simulink model "LUT_liver_pancreas_25"  (R2023b)
settings: Solver=FixedStepAuto  StartTime=0  StopTime=10.1  FixedStep=Timegap  RelTol=1e-3
model workspace (MAT data in the model file):
  T1_input = 1.34
(part 1 of 3)
settings Model: Creator=ppxmr2  LastModifiedBy=ppxmr2

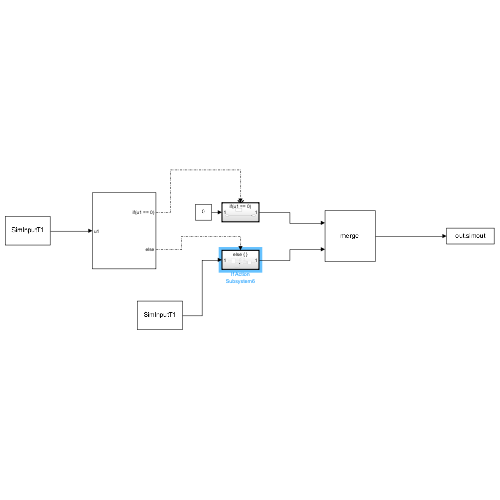
[thumbnail: Simulink's stored preview of the top-level diagram]
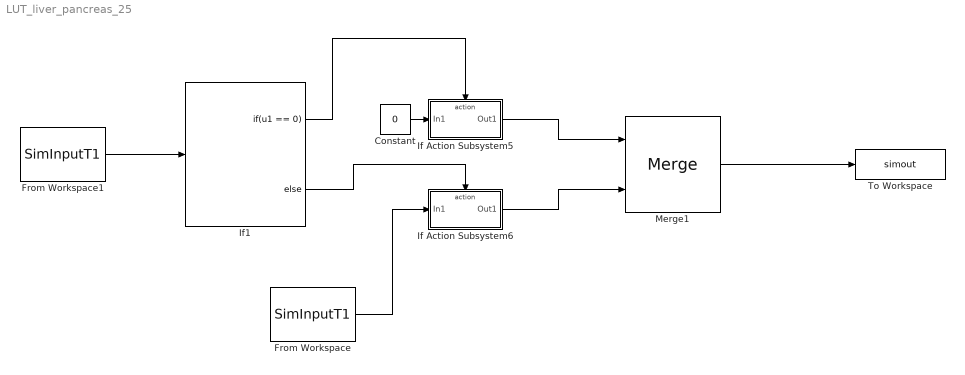
== system LUT_liver_pancreas_25 ==
  Constant : Constant  Value=0
  From Workspace : FromWorkspace  VariableName=SimInputT1  Interpolate=off  OutputAfterFinalValue=Setting to zero
  From Workspace1 : FromWorkspace  VariableName=SimInputT1  Interpolate=off  OutputAfterFinalValue=Setting to zero
  If Action Subsystem5 : Subsystem  TreatAsAtomicUnit=on
  If Action Subsystem6 : Subsystem  TreatAsAtomicUnit=on
  If1 : If  IfExpression=u1 == 0
  Merge1 : Merge
  To Workspace : ToWorkspace  VariableName=simout
  wires:
  From Workspace1/1 -> If1/1
  If1/1 -> If Action Subsystem5/Action
  If1/2 -> If Action Subsystem6/Action
  Constant/1 -> If Action Subsystem5/1(In1)
  If Action Subsystem5/1(Out1) -> Merge1/1
  If Action Subsystem6/1(Out1) -> Merge1/2
  Merge1/1 -> To Workspace/1
  From Workspace/1 -> If Action Subsystem6/1(In1)

== system LUT_liver_pancreas_25/If Action Subsystem5 ==
  In1 : Inport
  Action Port : ActionPort  ActionPortLabel=if(u1 == 0)
  Out1 : Outport
  wires:
  In1/1 -> Out1/1

== system LUT_liver_pancreas_25/If Action Subsystem6 ==
  In1 : Inport
  Action Port : ActionPort  ActionPortLabel=else
  From Workspace1 : FromWorkspace  VariableName=SimInputHR  Interpolate=off  OutputAfterFinalValue=Setting to zero
  If : If  IfExpression=u1 >= 1.495  ElseIfExpressions=u1 >= 0.995
  If Action Subsystem1 : Subsystem  TreatAsAtomicUnit=on
  If Action Subsystem2 : Subsystem  TreatAsAtomicUnit=on
  If Action Subsystem3 : Subsystem  TreatAsAtomicUnit=on
  Merge : Merge  Inputs=3
  Out1 : Outport
  wires:
  Merge/1 -> Out1/1
  From Workspace1/1 -> If/1
  If Action Subsystem1/1(Out1) -> Merge/2
  If Action Subsystem3/1(Out1) -> Merge/3
  In1/1 -> If Action Subsystem2/1(In1), If Action Subsystem1/1(In1), If Action Subsystem3/1(In1)
  If/1 -> If Action Subsystem2/Action
  If/2 -> If Action Subsystem1/Action
  If/3 -> If Action Subsystem3/Action
  If Action Subsystem2/1(Out1) -> Merge/1

== system LUT_liver_pancreas_25/If Action Subsystem6/If Action Subsystem1 ==
  In1 : Inport
  Action Port : ActionPort  ActionPortLabel=elseif(u1 >= 0.995)
  From Workspace2 : FromWorkspace  VariableName=SimInputHR  Interpolate=off  OutputAfterFinalValue=Setting to zero
  If Action Subsystem5 : Subsystem  TreatAsAtomicUnit=on
  If Action Subsystem6 : Subsystem  TreatAsAtomicUnit=on
  If Action Subsystem7 : Subsystem  TreatAsAtomicUnit=on
  If Action Subsystem8 : Subsystem  TreatAsAtomicUnit=on
  If Action Subsystem9 : Subsystem  TreatAsAtomicUnit=on
  If1 : If  IfExpression=u1 >= 1.395  ElseIfExpressions=u1 >= 1.295, u1 >= 1.195, u1 >= 1.095
  Merge1 : Merge  Inputs=5
  Out1 : Outport
  wires:
  In1/1 -> If Action Subsystem7/1(In2), If Action Subsystem8/1(In1), If Action Subsystem9/1(In1), If Action Subsystem5/1(In1), If Action Subsystem6/1(In1)
  From Workspace2/1 -> If1/1
  If Action Subsystem9/1(Out1) -> Merge1/1
  If Action Subsystem6/1(Out1) -> Merge1/5
  If Action Subsystem8/1(Out1) -> Merge1/2
  If Action Subsystem5/1(Out1) -> Merge1/4
  If1/4 -> If Action Subsystem5/Action
  If1/2 -> If Action Subsystem8/Action
  If1/3 -> If Action Subsystem7/Action
  If Action Subsystem7/1(Out2) -> Merge1/3
  If1/5 -> If Action Subsystem6/Action
  If1/1 -> If Action Subsystem9/Action
  Merge1/1 -> Out1/1

== system LUT_liver_pancreas_25/If Action Subsystem6/If Action Subsystem2 ==
  In1 : Inport
  Action Port : ActionPort  ActionPortLabel=if(u1 >= 1.495)
  From Workspace2 : FromWorkspace  VariableName=SimInputHR  Interpolate=off  OutputAfterFinalValue=Setting to zero
  If Action Subsystem5 : Subsystem  TreatAsAtomicUnit=on
  If Action Subsystem6 : Subsystem  TreatAsAtomicUnit=on
  If Action Subsystem7 : Subsystem  TreatAsAtomicUnit=on
  If Action Subsystem8 : Subsystem  TreatAsAtomicUnit=on
  If Action Subsystem9 : Subsystem  TreatAsAtomicUnit=on
  If1 : If  IfExpression=u1 >= 1.895  ElseIfExpressions=u1 >= 1.795, u1 >= 1.695, u1 >= 1.595
  Merge1 : Merge  Inputs=5
  Out1 : Outport
  wires:
  In1/1 -> If Action Subsystem9/1(In1), If Action Subsystem8/1(In1), If Action Subsystem7/1(In1), If Action Subsystem5/1(In1), If Action Subsystem6/1(In1)
  From Workspace2/1 -> If1/1
  If Action Subsystem9/1(Out1) -> Merge1/1
  If1/4 -> If Action Subsystem5/Action
  If1/2 -> If Action Subsystem8/Action
  If1/3 -> If Action Subsystem7/Action
  If1/5 -> If Action Subsystem6/Action
  If1/1 -> If Action Subsystem9/Action
  Merge1/1 -> Out1/1
  If Action Subsystem8/1(Out1) -> Merge1/2
  If Action Subsystem7/1(Out1) -> Merge1/3
  If Action Subsystem6/1(Out1) -> Merge1/5
  If Action Subsystem5/1(Out1) -> Merge1/4

== system LUT_liver_pancreas_25/If Action Subsystem6/If Action Subsystem3 ==
  In1 : Inport
  Action Port : ActionPort  ActionPortLabel=else
  From Workspace2 : FromWorkspace  VariableName=SimInputHR  Interpolate=off  OutputAfterFinalValue=Setting to zero
  If Action Subsystem5 : Subsystem  TreatAsAtomicUnit=on
  If Action Subsystem6 : Subsystem  TreatAsAtomicUnit=on
  If Action Subsystem7 : Subsystem  TreatAsAtomicUnit=on
  If Action Subsystem8 : Subsystem  TreatAsAtomicUnit=on
  If Action Subsystem9 : Subsystem  TreatAsAtomicUnit=on
  If1 : If  IfExpression=u1 >= 0.895  ElseIfExpressions=u1 >= 0.795, u1 >= 0.695, u1 >= 0595
  Merge1 : Merge  Inputs=5
  Out1 : Outport
  wires:
  In1/1 -> If Action Subsystem8/1(In1), If Action Subsystem9/1(In2), If Action Subsystem7/1(In1), If Action Subsystem5/1(In1), If Action Subsystem6/1(In1)
  From Workspace2/1 -> If1/1
  If Action Subsystem9/1(Out2) -> Merge1/1
  If Action Subsystem6/1(Out1) -> Merge1/5
  If Action Subsystem8/1(Out1) -> Merge1/2
  If Action Subsystem5/1(Out1) -> Merge1/4
  If1/4 -> If Action Subsystem5/Action
  If1/2 -> If Action Subsystem8/Action
  If1/3 -> If Action Subsystem7/Action
  If Action Subsystem7/1(Out1) -> Merge1/3
  If1/5 -> If Action Subsystem6/Action
  If1/1 -> If Action Subsystem9/Action
  Merge1/1 -> Out1/1

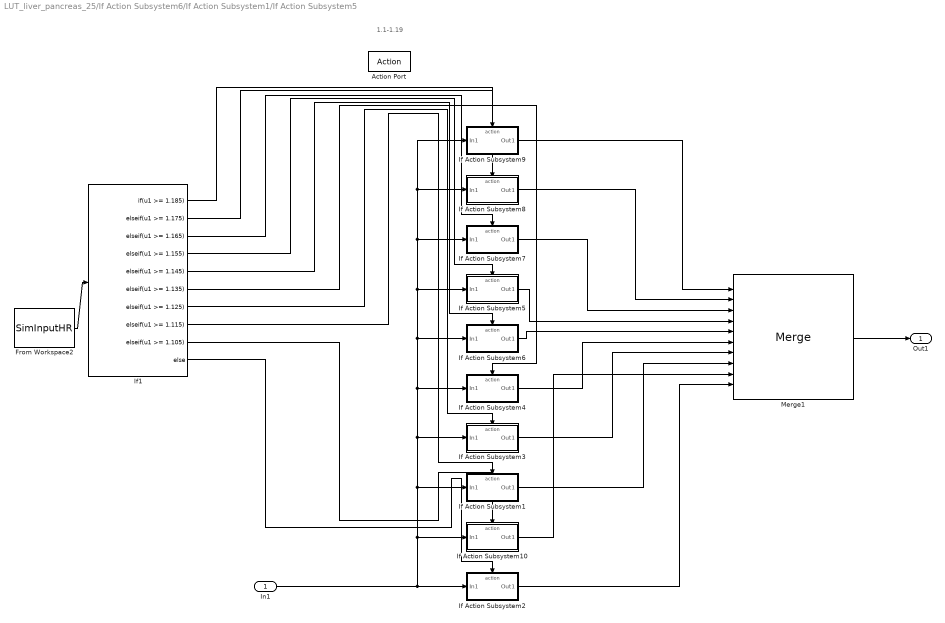
== system LUT_liver_pancreas_25/If Action Subsystem6/If Action Subsystem1/If Action Subsystem5 ==
  note: 1.1-1.19
  In1 : Inport
  Action Port : ActionPort  ActionPortLabel=elseif( u1 >= 1.095)
  From Workspace2 : FromWorkspace  VariableName=SimInputHR  Interpolate=off  OutputAfterFinalValue=Setting to zero
  If Action Subsystem1 : Subsystem  TreatAsAtomicUnit=on
  If Action Subsystem10 : Subsystem  TreatAsAtomicUnit=on
  If Action Subsystem2 : Subsystem  TreatAsAtomicUnit=on
  If Action Subsystem3 : Subsystem  TreatAsAtomicUnit=on
  If Action Subsystem4 : Subsystem  TreatAsAtomicUnit=on
  If Action Subsystem5 : Subsystem  TreatAsAtomicUnit=on
  If Action Subsystem6 : Subsystem  TreatAsAtomicUnit=on
  If Action Subsystem7 : Subsystem  TreatAsAtomicUnit=on
  If Action Subsystem8 : Subsystem  TreatAsAtomicUnit=on
  If Action Subsystem9 : Subsystem  TreatAsAtomicUnit=on
  If1 : If  IfExpression=u1 >= 1.185  ElseIfExpressions=u1 >= 1.175, u1 >= 1.165, u1 >= 1.155, u1 >= 1.145, u1 >= 1.135, u1 >= 1.125, u1 >= 1.115, u1 >= 1.105
  Merge1 : Merge  Inputs=10
  Out1 : Outport
  wires:
  If1/10 -> If Action Subsystem2/Action
  If Action Subsystem4/1(Out1) -> Merge1/6
  From Workspace2/1 -> If1/1
  If Action Subsystem6/1(Out1) -> Merge1/5
  Merge1/1 -> Out1/1
  If1/8 -> If Action Subsystem1/Action
  If Action Subsystem3/1(Out1) -> Merge1/7
  In1/1 -> If Action Subsystem1/1(In1), If Action Subsystem3/1(In1), If Action Subsystem4/1(In1), If Action Subsystem7/1(In1), If Action Subsystem8/1(In1), If Action Subsystem9/1(In1), If Action Subsystem5/1(In1), If Action Subsystem6/1(In1), If Action Subsystem10/1(In1), If Action Subsystem2/1(In1)
  If1/6 -> If Action Subsystem4/Action
  If Action Subsystem1/1(Out1) -> Merge1/8
  If1/4 -> If Action Subsystem5/Action
  If Action Subsystem8/1(Out1) -> Merge1/2
  If1/5 -> If Action Subsystem6/Action
  If Action Subsystem7/1(Out1) -> Merge1/3
  If1/3 -> If Action Subsystem7/Action
  If1/7 -> If Action Subsystem3/Action
  If Action Subsystem5/1(Out1) -> Merge1/4
  If Action Subsystem2/1(Out1) -> Merge1/10
  If1/2 -> If Action Subsystem8/Action
  If1/1 -> If Action Subsystem9/Action
  If Action Subsystem9/1(Out1) -> Merge1/1
  If1/9 -> If Action Subsystem10/Action
  If Action Subsystem10/1(Out1) -> Merge1/9

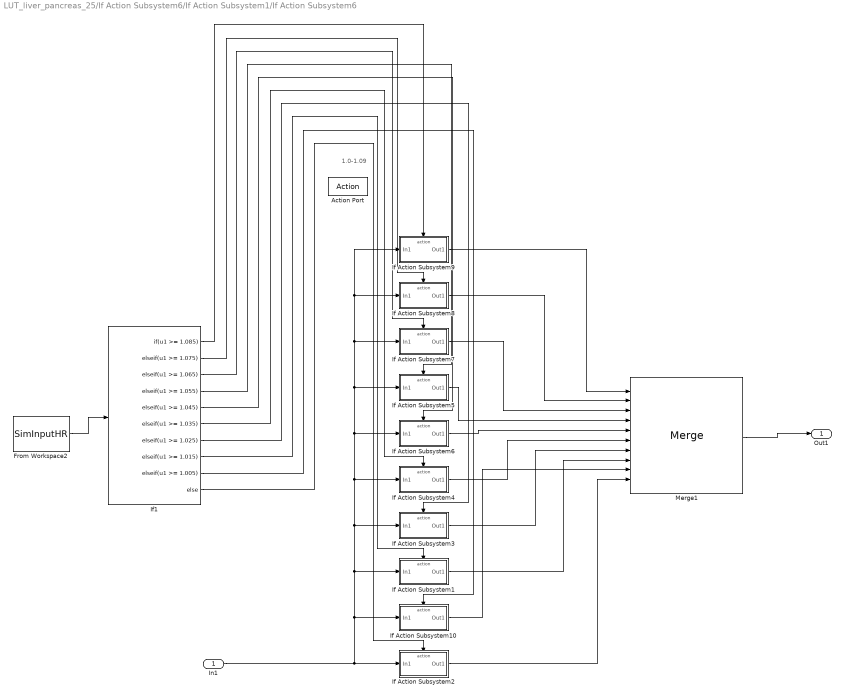
== system LUT_liver_pancreas_25/If Action Subsystem6/If Action Subsystem1/If Action Subsystem6 ==
  note: 1.0-1.09
  In1 : Inport
  Action Port : ActionPort  ActionPortLabel=else
  From Workspace2 : FromWorkspace  VariableName=SimInputHR  Interpolate=off  OutputAfterFinalValue=Setting to zero
  If Action Subsystem1 : Subsystem  TreatAsAtomicUnit=on
  If Action Subsystem10 : Subsystem  TreatAsAtomicUnit=on
  If Action Subsystem2 : Subsystem  TreatAsAtomicUnit=on
  If Action Subsystem3 : Subsystem  TreatAsAtomicUnit=on
  If Action Subsystem4 : Subsystem  TreatAsAtomicUnit=on
  If Action Subsystem5 : Subsystem  TreatAsAtomicUnit=on
  If Action Subsystem6 : Subsystem  TreatAsAtomicUnit=on
  If Action Subsystem7 : Subsystem  TreatAsAtomicUnit=on
  If Action Subsystem8 : Subsystem  TreatAsAtomicUnit=on
  If Action Subsystem9 : Subsystem  TreatAsAtomicUnit=on
  If1 : If  IfExpression=u1 >= 1.085  ElseIfExpressions=u1 >= 1.075, u1 >= 1.065, u1 >= 1.055, u1 >= 1.045, u1 >= 1.035, u1 >= 1.025, u1 >= 1.015, u1 >= 1.005
  Merge1 : Merge  Inputs=10
  Out1 : Outport
  wires:
  If1/10 -> If Action Subsystem2/Action
  If Action Subsystem4/1(Out1) -> Merge1/6
  From Workspace2/1 -> If1/1
  If Action Subsystem6/1(Out1) -> Merge1/5
  Merge1/1 -> Out1/1
  If1/8 -> If Action Subsystem1/Action
  If Action Subsystem3/1(Out1) -> Merge1/7
  In1/1 -> If Action Subsystem1/1(In1), If Action Subsystem3/1(In1), If Action Subsystem4/1(In1), If Action Subsystem7/1(In1), If Action Subsystem8/1(In1), If Action Subsystem9/1(In1), If Action Subsystem5/1(In1), If Action Subsystem6/1(In1), If Action Subsystem10/1(In1), If Action Subsystem2/1(In1)
  If1/6 -> If Action Subsystem4/Action
  If Action Subsystem1/1(Out1) -> Merge1/8
  If1/4 -> If Action Subsystem5/Action
  If Action Subsystem8/1(Out1) -> Merge1/2
  If1/5 -> If Action Subsystem6/Action
  If Action Subsystem7/1(Out1) -> Merge1/3
  If1/3 -> If Action Subsystem7/Action
  If1/7 -> If Action Subsystem3/Action
  If Action Subsystem5/1(Out1) -> Merge1/4
  If Action Subsystem2/1(Out1) -> Merge1/10
  If1/2 -> If Action Subsystem8/Action
  If1/1 -> If Action Subsystem9/Action
  If Action Subsystem9/1(Out1) -> Merge1/1
  If1/9 -> If Action Subsystem10/Action
  If Action Subsystem10/1(Out1) -> Merge1/9

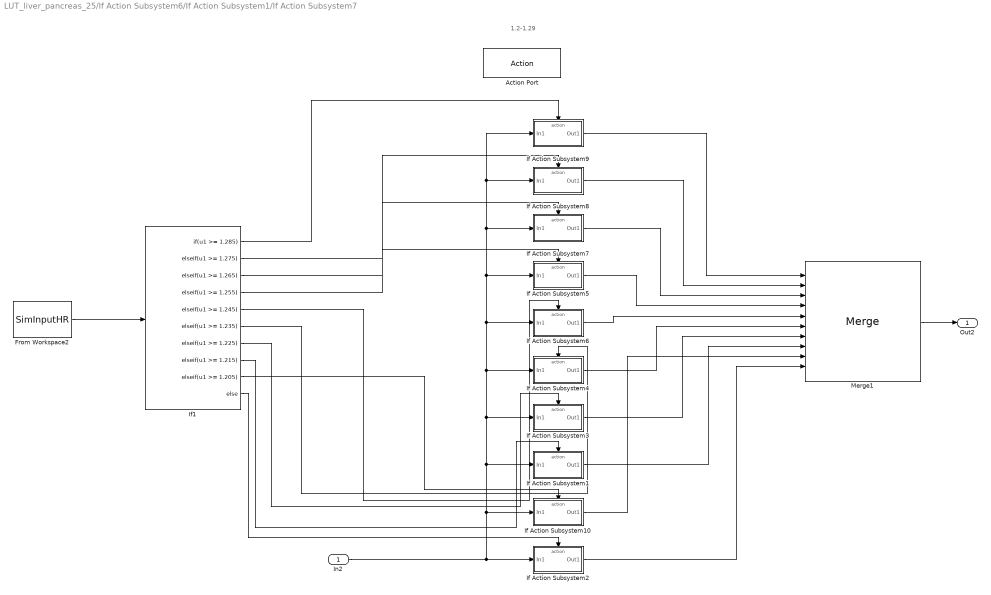
== system LUT_liver_pancreas_25/If Action Subsystem6/If Action Subsystem1/If Action Subsystem7 ==
  note: 1.2-1.29
  In2 : Inport
  Action Port : ActionPort  ActionPortLabel=elseif( u1 >= 1.195)
  From Workspace2 : FromWorkspace  VariableName=SimInputHR  Interpolate=off  OutputAfterFinalValue=Setting to zero
  If Action Subsystem1 : Subsystem  TreatAsAtomicUnit=on
  If Action Subsystem10 : Subsystem  TreatAsAtomicUnit=on
  If Action Subsystem2 : Subsystem  TreatAsAtomicUnit=on
  If Action Subsystem3 : Subsystem  TreatAsAtomicUnit=on
  If Action Subsystem4 : Subsystem  TreatAsAtomicUnit=on
  If Action Subsystem5 : Subsystem  TreatAsAtomicUnit=on
  If Action Subsystem6 : Subsystem  TreatAsAtomicUnit=on
  If Action Subsystem7 : Subsystem  TreatAsAtomicUnit=on
  If Action Subsystem8 : Subsystem  TreatAsAtomicUnit=on
  If Action Subsystem9 : Subsystem  TreatAsAtomicUnit=on
  If1 : If  IfExpression=u1 >= 1.285  ElseIfExpressions=u1 >= 1.275, u1 >= 1.265, u1 >= 1.255, u1 >= 1.245, u1 >= 1.235, u1 >= 1.225, u1 >= 1.215, u1 >= 1.205
  Merge1 : Merge  Inputs=10
  Out2 : Outport
  wires:
  If1/10 -> If Action Subsystem2/Action
  If Action Subsystem4/1(Out1) -> Merge1/6
  From Workspace2/1 -> If1/1
  If Action Subsystem6/1(Out1) -> Merge1/5
  Merge1/1 -> Out2/1
  If1/8 -> If Action Subsystem1/Action
  If Action Subsystem3/1(Out1) -> Merge1/7
  In2/1 -> If Action Subsystem1/1(In1), If Action Subsystem3/1(In1), If Action Subsystem4/1(In1), If Action Subsystem7/1(In1), If Action Subsystem8/1(In1), If Action Subsystem9/1(In1), If Action Subsystem5/1(In1), If Action Subsystem6/1(In1), If Action Subsystem10/1(In1), If Action Subsystem2/1(In1)
  If1/6 -> If Action Subsystem4/Action
  If Action Subsystem1/1(Out1) -> Merge1/8
  If1/4 -> If Action Subsystem5/Action
  If Action Subsystem8/1(Out1) -> Merge1/2
  If1/5 -> If Action Subsystem6/Action
  If Action Subsystem7/1(Out1) -> Merge1/3
  If1/3 -> If Action Subsystem7/Action
  If1/7 -> If Action Subsystem3/Action
  If Action Subsystem5/1(Out1) -> Merge1/4
  If Action Subsystem2/1(Out1) -> Merge1/10
  If1/2 -> If Action Subsystem8/Action
  If1/1 -> If Action Subsystem9/Action
  If Action Subsystem9/1(Out1) -> Merge1/1
  If Action Subsystem10/1(Out1) -> Merge1/9
  If1/9 -> If Action Subsystem10/Action

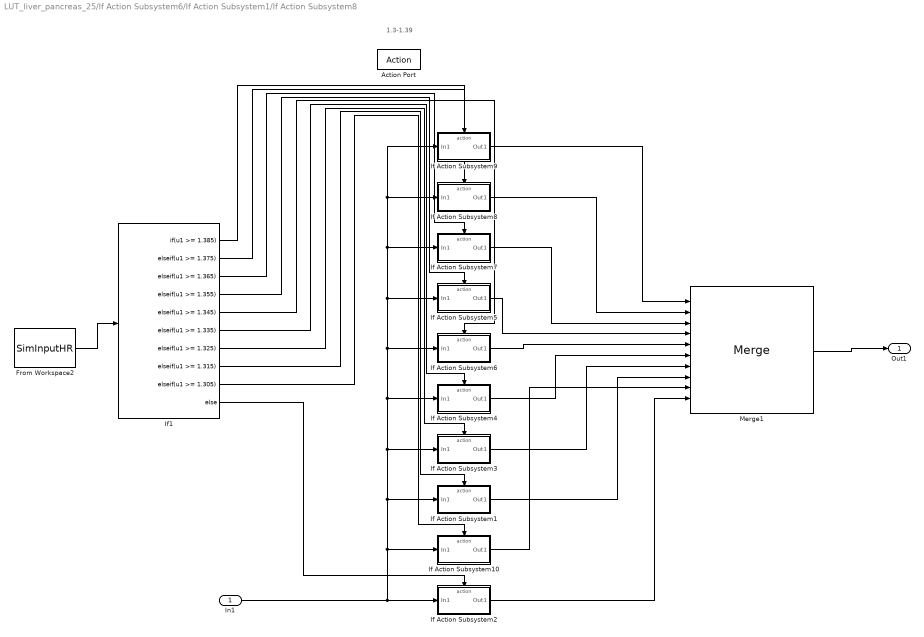
== system LUT_liver_pancreas_25/If Action Subsystem6/If Action Subsystem1/If Action Subsystem8 ==
  note: 1.3-1.39
  In1 : Inport
  Action Port : ActionPort  ActionPortLabel=elseif(u1 >= 1.295)
  From Workspace2 : FromWorkspace  VariableName=SimInputHR  Interpolate=off  OutputAfterFinalValue=Setting to zero
  If Action Subsystem1 : Subsystem  TreatAsAtomicUnit=on
  If Action Subsystem10 : Subsystem  TreatAsAtomicUnit=on
  If Action Subsystem2 : Subsystem  TreatAsAtomicUnit=on
  If Action Subsystem3 : Subsystem  TreatAsAtomicUnit=on
  If Action Subsystem4 : Subsystem  TreatAsAtomicUnit=on
  If Action Subsystem5 : Subsystem  TreatAsAtomicUnit=on
  If Action Subsystem6 : Subsystem  TreatAsAtomicUnit=on
  If Action Subsystem7 : Subsystem  TreatAsAtomicUnit=on
  If Action Subsystem8 : Subsystem  TreatAsAtomicUnit=on
  If Action Subsystem9 : Subsystem  TreatAsAtomicUnit=on
  If1 : If  IfExpression=u1 >= 1.385  ElseIfExpressions=u1 >= 1.375, u1 >= 1.365, u1 >= 1.355, u1 >= 1.345, u1 >= 1.335, u1 >= 1.325, u1 >= 1.315, u1 >= 1.305
  Merge1 : Merge  Inputs=10
  Out1 : Outport
  wires:
  If1/10 -> If Action Subsystem2/Action
  If Action Subsystem4/1(Out1) -> Merge1/6
  From Workspace2/1 -> If1/1
  If Action Subsystem6/1(Out1) -> Merge1/5
  Merge1/1 -> Out1/1
  If1/8 -> If Action Subsystem1/Action
  If Action Subsystem3/1(Out1) -> Merge1/7
  In1/1 -> If Action Subsystem1/1(In1), If Action Subsystem3/1(In1), If Action Subsystem4/1(In1), If Action Subsystem7/1(In1), If Action Subsystem8/1(In1), If Action Subsystem9/1(In1), If Action Subsystem5/1(In1), If Action Subsystem6/1(In1), If Action Subsystem10/1(In1), If Action Subsystem2/1(In1)
  If1/6 -> If Action Subsystem4/Action
  If Action Subsystem1/1(Out1) -> Merge1/8
  If1/4 -> If Action Subsystem5/Action
  If Action Subsystem8/1(Out1) -> Merge1/2
  If1/5 -> If Action Subsystem6/Action
  If Action Subsystem7/1(Out1) -> Merge1/3
  If1/3 -> If Action Subsystem7/Action
  If1/7 -> If Action Subsystem3/Action
  If Action Subsystem5/1(Out1) -> Merge1/4
  If Action Subsystem2/1(Out1) -> Merge1/10
  If1/2 -> If Action Subsystem8/Action
  If1/1 -> If Action Subsystem9/Action
  If Action Subsystem9/1(Out1) -> Merge1/1
  If1/9 -> If Action Subsystem10/Action
  If Action Subsystem10/1(Out1) -> Merge1/9

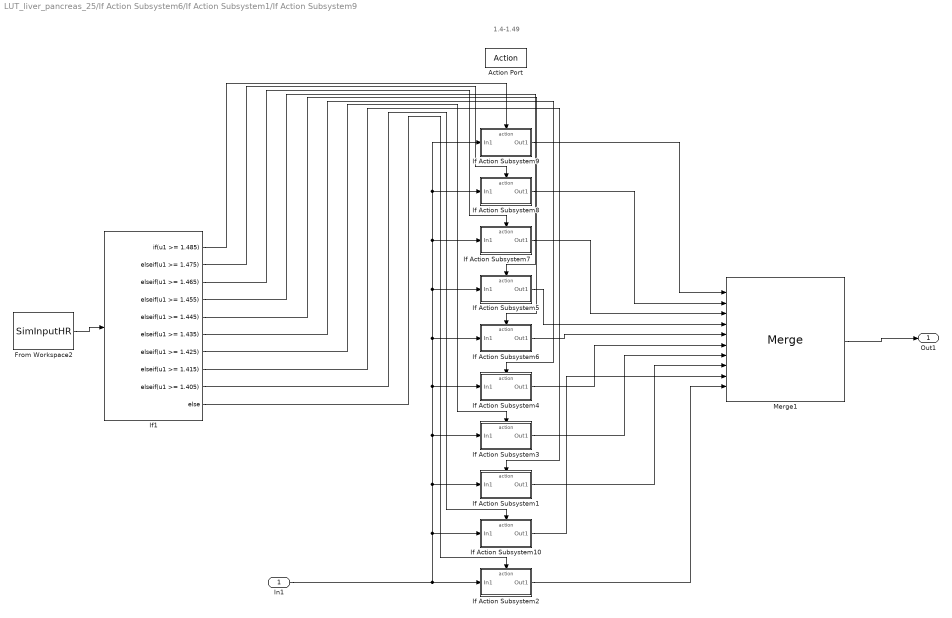
== system LUT_liver_pancreas_25/If Action Subsystem6/If Action Subsystem1/If Action Subsystem9 ==
  note: 1.4-1.49
  In1 : Inport
  Action Port : ActionPort  ActionPortLabel=if(u1 >= 1.395)
  From Workspace2 : FromWorkspace  VariableName=SimInputHR  Interpolate=off  OutputAfterFinalValue=Setting to zero
  If Action Subsystem1 : Subsystem  TreatAsAtomicUnit=on
  If Action Subsystem10 : Subsystem  TreatAsAtomicUnit=on
  If Action Subsystem2 : Subsystem  TreatAsAtomicUnit=on
  If Action Subsystem3 : Subsystem  TreatAsAtomicUnit=on
  If Action Subsystem4 : Subsystem  TreatAsAtomicUnit=on
  If Action Subsystem5 : Subsystem  TreatAsAtomicUnit=on
  If Action Subsystem6 : Subsystem  TreatAsAtomicUnit=on
  If Action Subsystem7 : Subsystem  TreatAsAtomicUnit=on
  If Action Subsystem8 : Subsystem  TreatAsAtomicUnit=on
  If Action Subsystem9 : Subsystem  TreatAsAtomicUnit=on
  If1 : If  IfExpression=u1 >= 1.485  ElseIfExpressions=u1 >= 1.475, u1 >= 1.465, u1 >= 1.455, u1 >= 1.445, u1 >= 1.435, u1 >= 1.425, u1 >= 1.415, u1 >= 1.405
  Merge1 : Merge  Inputs=10
  Out1 : Outport
  wires:
  If1/10 -> If Action Subsystem2/Action
  If Action Subsystem4/1(Out1) -> Merge1/6
  From Workspace2/1 -> If1/1
  If Action Subsystem6/1(Out1) -> Merge1/5
  Merge1/1 -> Out1/1
  If1/8 -> If Action Subsystem1/Action
  If Action Subsystem3/1(Out1) -> Merge1/7
  In1/1 -> If Action Subsystem10/1(In1), If Action Subsystem1/1(In1), If Action Subsystem3/1(In1), If Action Subsystem4/1(In1), If Action Subsystem7/1(In1), If Action Subsystem8/1(In1), If Action Subsystem9/1(In1), If Action Subsystem5/1(In1), If Action Subsystem6/1(In1), If Action Subsystem2/1(In1)
  If1/6 -> If Action Subsystem4/Action
  If Action Subsystem1/1(Out1) -> Merge1/8
  If1/4 -> If Action Subsystem5/Action
  If Action Subsystem8/1(Out1) -> Merge1/2
  If1/5 -> If Action Subsystem6/Action
  If Action Subsystem7/1(Out1) -> Merge1/3
  If1/3 -> If Action Subsystem7/Action
  If1/7 -> If Action Subsystem3/Action
  If Action Subsystem5/1(Out1) -> Merge1/4
  If Action Subsystem2/1(Out1) -> Merge1/10
  If1/2 -> If Action Subsystem8/Action
  If1/1 -> If Action Subsystem9/Action
  If Action Subsystem9/1(Out1) -> Merge1/1
  If1/9 -> If Action Subsystem10/Action
  If Action Subsystem10/1(Out1) -> Merge1/9

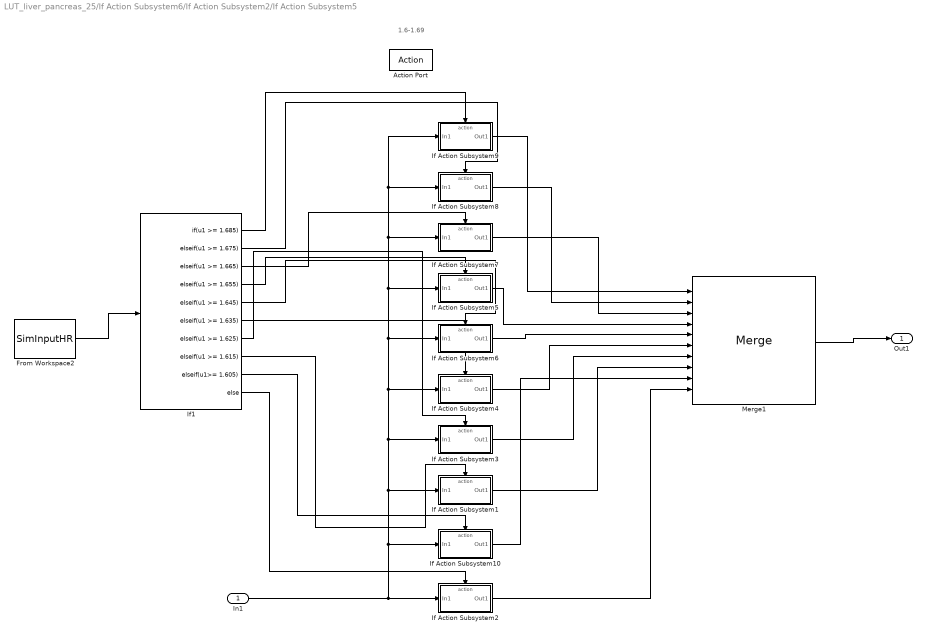
== system LUT_liver_pancreas_25/If Action Subsystem6/If Action Subsystem2/If Action Subsystem5 ==
  note: 1.6-1.69
  In1 : Inport
  Action Port : ActionPort  ActionPortLabel=elseif( u1 >= 1.595)
  From Workspace2 : FromWorkspace  VariableName=SimInputHR  Interpolate=off  OutputAfterFinalValue=Setting to zero
  If Action Subsystem1 : Subsystem  TreatAsAtomicUnit=on
  If Action Subsystem10 : Subsystem  TreatAsAtomicUnit=on
  If Action Subsystem2 : Subsystem  TreatAsAtomicUnit=on
  If Action Subsystem3 : Subsystem  TreatAsAtomicUnit=on
  If Action Subsystem4 : Subsystem  TreatAsAtomicUnit=on
  If Action Subsystem5 : Subsystem  TreatAsAtomicUnit=on
  If Action Subsystem6 : Subsystem  TreatAsAtomicUnit=on
  If Action Subsystem7 : Subsystem  TreatAsAtomicUnit=on
  If Action Subsystem8 : Subsystem  TreatAsAtomicUnit=on
  If Action Subsystem9 : Subsystem  TreatAsAtomicUnit=on
  If1 : If  IfExpression=u1 >= 1.685  ElseIfExpressions=u1 >= 1.675, u1 >= 1.665, u1 >= 1.655, u1 >= 1.645, u1 >= 1.635, u1 >= 1.625, u1 >= 1.615, u1>= 1.605
  Merge1 : Merge  Inputs=10
  Out1 : Outport
  wires:
  If1/2 -> If Action Subsystem8/Action
  If Action Subsystem5/1(Out1) -> Merge1/4
  If1/3 -> If Action Subsystem7/Action
  If Action Subsystem9/1(Out1) -> Merge1/1
  If1/7 -> If Action Subsystem3/Action
  If1/5 -> If Action Subsystem6/Action
  If1/1 -> If Action Subsystem9/Action
  If Action Subsystem4/1(Out1) -> Merge1/6
  If1/10 -> If Action Subsystem2/Action
  If Action Subsystem8/1(Out1) -> Merge1/2
  If1/4 -> If Action Subsystem5/Action
  In1/1 -> If Action Subsystem10/1(In1), If Action Subsystem1/1(In1), If Action Subsystem3/1(In1), If Action Subsystem4/1(In1), If Action Subsystem7/1(In1), If Action Subsystem8/1(In1), If Action Subsystem9/1(In1), If Action Subsystem5/1(In1), If Action Subsystem6/1(In1), If Action Subsystem2/1(In1)
  If Action Subsystem1/1(Out1) -> Merge1/8
  If Action Subsystem2/1(Out1) -> Merge1/10
  If1/8 -> If Action Subsystem1/Action
  If Action Subsystem3/1(Out1) -> Merge1/7
  If1/6 -> If Action Subsystem4/Action
  From Workspace2/1 -> If1/1
  Merge1/1 -> Out1/1
  If Action Subsystem6/1(Out1) -> Merge1/5
  If Action Subsystem7/1(Out1) -> Merge1/3
  If1/9 -> If Action Subsystem10/Action
  If Action Subsystem10/1(Out1) -> Merge1/9

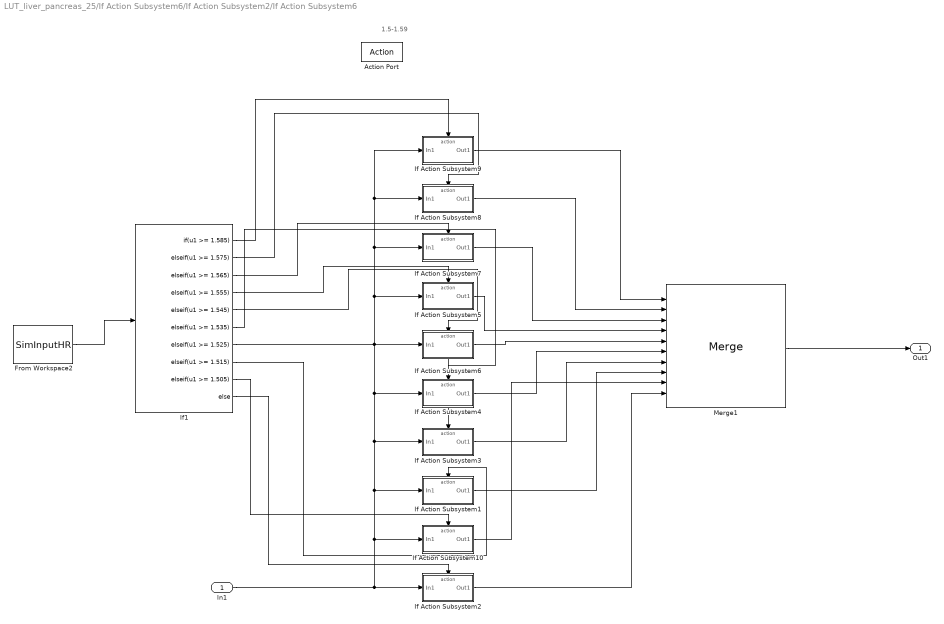
== system LUT_liver_pancreas_25/If Action Subsystem6/If Action Subsystem2/If Action Subsystem6 ==
  note: 1.5-1.59
  In1 : Inport
  Action Port : ActionPort  ActionPortLabel=else
  From Workspace2 : FromWorkspace  VariableName=SimInputHR  Interpolate=off  OutputAfterFinalValue=Setting to zero
  If Action Subsystem1 : Subsystem  TreatAsAtomicUnit=on
  If Action Subsystem10 : Subsystem  TreatAsAtomicUnit=on
  If Action Subsystem2 : Subsystem  TreatAsAtomicUnit=on
  If Action Subsystem3 : Subsystem  TreatAsAtomicUnit=on
  If Action Subsystem4 : Subsystem  TreatAsAtomicUnit=on
  If Action Subsystem5 : Subsystem  TreatAsAtomicUnit=on
  If Action Subsystem6 : Subsystem  TreatAsAtomicUnit=on
  If Action Subsystem7 : Subsystem  TreatAsAtomicUnit=on
  If Action Subsystem8 : Subsystem  TreatAsAtomicUnit=on
  If Action Subsystem9 : Subsystem  TreatAsAtomicUnit=on
  If1 : If  IfExpression=u1 >= 1.585  ElseIfExpressions=u1 >= 1.575, u1 >= 1.565, u1 >= 1.555, u1 >= 1.545, u1 >= 1.535, u1 >= 1.525, u1 >= 1.515, u1 >= 1.505
  Merge1 : Merge  Inputs=10
  Out1 : Outport
  wires:
  If1/2 -> If Action Subsystem8/Action
  If Action Subsystem5/1(Out1) -> Merge1/4
  If1/3 -> If Action Subsystem7/Action
  If Action Subsystem9/1(Out1) -> Merge1/1
  If1/7 -> If Action Subsystem3/Action
  If1/5 -> If Action Subsystem6/Action
  If1/1 -> If Action Subsystem9/Action
  If Action Subsystem4/1(Out1) -> Merge1/6
  If1/10 -> If Action Subsystem2/Action
  If Action Subsystem8/1(Out1) -> Merge1/2
  If1/4 -> If Action Subsystem5/Action
  In1/1 -> If Action Subsystem10/1(In1), If Action Subsystem1/1(In1), If Action Subsystem3/1(In1), If Action Subsystem4/1(In1), If Action Subsystem7/1(In1), If Action Subsystem8/1(In1), If Action Subsystem9/1(In1), If Action Subsystem5/1(In1), If Action Subsystem6/1(In1), If Action Subsystem2/1(In1)
  If Action Subsystem1/1(Out1) -> Merge1/8
  If Action Subsystem2/1(Out1) -> Merge1/10
  If1/8 -> If Action Subsystem1/Action
  If Action Subsystem3/1(Out1) -> Merge1/7
  If1/6 -> If Action Subsystem4/Action
  From Workspace2/1 -> If1/1
  Merge1/1 -> Out1/1
  If Action Subsystem6/1(Out1) -> Merge1/5
  If Action Subsystem7/1(Out1) -> Merge1/3
  If1/9 -> If Action Subsystem10/Action
  If Action Subsystem10/1(Out1) -> Merge1/9

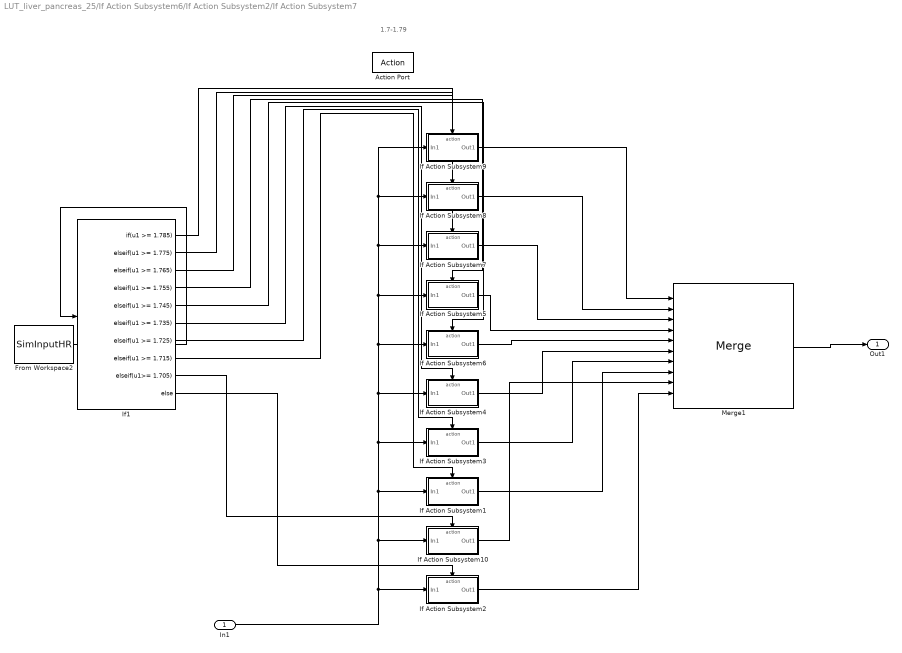
== system LUT_liver_pancreas_25/If Action Subsystem6/If Action Subsystem2/If Action Subsystem7 ==
  note: 1.7-1.79
  In1 : Inport
  Action Port : ActionPort  ActionPortLabel=elseif( u1 >= 1.695)
  From Workspace2 : FromWorkspace  VariableName=SimInputHR  Interpolate=off  OutputAfterFinalValue=Setting to zero
  If Action Subsystem1 : Subsystem  TreatAsAtomicUnit=on
  If Action Subsystem10 : Subsystem  TreatAsAtomicUnit=on
  If Action Subsystem2 : Subsystem  TreatAsAtomicUnit=on
  If Action Subsystem3 : Subsystem  TreatAsAtomicUnit=on
  If Action Subsystem4 : Subsystem  TreatAsAtomicUnit=on
  If Action Subsystem5 : Subsystem  TreatAsAtomicUnit=on
  If Action Subsystem6 : Subsystem  TreatAsAtomicUnit=on
  If Action Subsystem7 : Subsystem  TreatAsAtomicUnit=on
  If Action Subsystem8 : Subsystem  TreatAsAtomicUnit=on
  If Action Subsystem9 : Subsystem  TreatAsAtomicUnit=on
  If1 : If  IfExpression=u1 >= 1.785  ElseIfExpressions=u1 >= 1.775, u1 >= 1.765, u1 >= 1.755, u1 >= 1.745, u1 >= 1.735, u1 >= 1.725, u1 >= 1.715, u1>= 1.705
  Merge1 : Merge  Inputs=10
  Out1 : Outport
  wires:
  If1/2 -> If Action Subsystem8/Action
  If Action Subsystem5/1(Out1) -> Merge1/4
  If1/3 -> If Action Subsystem7/Action
  If Action Subsystem9/1(Out1) -> Merge1/1
  If1/7 -> If Action Subsystem3/Action
  If1/5 -> If Action Subsystem6/Action
  If1/1 -> If Action Subsystem9/Action
  If Action Subsystem4/1(Out1) -> Merge1/6
  If1/10 -> If Action Subsystem2/Action
  If Action Subsystem8/1(Out1) -> Merge1/2
  If1/4 -> If Action Subsystem5/Action
  In1/1 -> If Action Subsystem10/1(In1), If Action Subsystem1/1(In1), If Action Subsystem3/1(In1), If Action Subsystem4/1(In1), If Action Subsystem7/1(In1), If Action Subsystem8/1(In1), If Action Subsystem9/1(In1), If Action Subsystem5/1(In1), If Action Subsystem6/1(In1), If Action Subsystem2/1(In1)
  If Action Subsystem1/1(Out1) -> Merge1/8
  If Action Subsystem2/1(Out1) -> Merge1/10
  If1/8 -> If Action Subsystem1/Action
  If Action Subsystem3/1(Out1) -> Merge1/7
  If1/6 -> If Action Subsystem4/Action
  From Workspace2/1 -> If1/1
  Merge1/1 -> Out1/1
  If Action Subsystem6/1(Out1) -> Merge1/5
  If Action Subsystem7/1(Out1) -> Merge1/3
  If Action Subsystem10/1(Out1) -> Merge1/9
  If1/9 -> If Action Subsystem10/Action

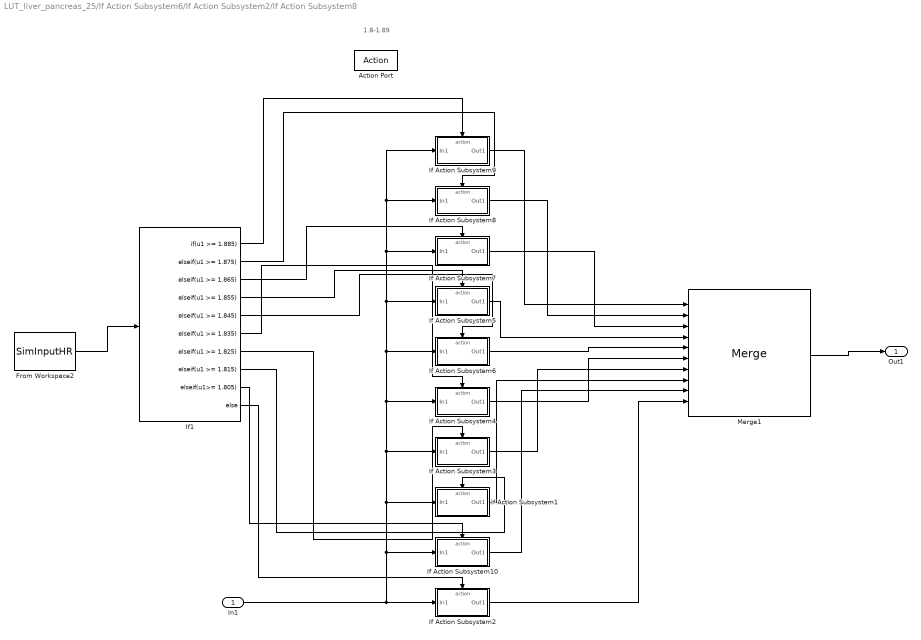
== system LUT_liver_pancreas_25/If Action Subsystem6/If Action Subsystem2/If Action Subsystem8 ==
  note: 1.8-1.89
  In1 : Inport
  Action Port : ActionPort  ActionPortLabel=elseif(u1 >= 1.795)
  From Workspace2 : FromWorkspace  VariableName=SimInputHR  Interpolate=off  OutputAfterFinalValue=Setting to zero
  If Action Subsystem1 : Subsystem  TreatAsAtomicUnit=on
  If Action Subsystem10 : Subsystem  TreatAsAtomicUnit=on
  If Action Subsystem2 : Subsystem  TreatAsAtomicUnit=on
  If Action Subsystem3 : Subsystem  TreatAsAtomicUnit=on
  If Action Subsystem4 : Subsystem  TreatAsAtomicUnit=on
  If Action Subsystem5 : Subsystem  TreatAsAtomicUnit=on
  If Action Subsystem6 : Subsystem  TreatAsAtomicUnit=on
  If Action Subsystem7 : Subsystem  TreatAsAtomicUnit=on
  If Action Subsystem8 : Subsystem  TreatAsAtomicUnit=on
  If Action Subsystem9 : Subsystem  TreatAsAtomicUnit=on
  If1 : If  IfExpression=u1 >= 1.885  ElseIfExpressions=u1 >= 1.875, u1 >= 1.865, u1 >= 1.855, u1 >= 1.845, u1 >= 1.835, u1 >= 1.825, u1 >= 1.815, u1>= 1.805
  Merge1 : Merge  Inputs=10
  Out1 : Outport
  wires:
  If1/2 -> If Action Subsystem8/Action
  If Action Subsystem5/1(Out1) -> Merge1/4
  If1/3 -> If Action Subsystem7/Action
  If Action Subsystem9/1(Out1) -> Merge1/1
  If1/7 -> If Action Subsystem3/Action
  If1/5 -> If Action Subsystem6/Action
  If1/1 -> If Action Subsystem9/Action
  If Action Subsystem4/1(Out1) -> Merge1/6
  If1/10 -> If Action Subsystem2/Action
  If Action Subsystem8/1(Out1) -> Merge1/2
  If1/4 -> If Action Subsystem5/Action
  In1/1 -> If Action Subsystem10/1(In1), If Action Subsystem1/1(In1), If Action Subsystem3/1(In1), If Action Subsystem4/1(In1), If Action Subsystem7/1(In1), If Action Subsystem8/1(In1), If Action Subsystem9/1(In1), If Action Subsystem5/1(In1), If Action Subsystem6/1(In1), If Action Subsystem2/1(In1)
  If Action Subsystem1/1(Out1) -> Merge1/8
  If Action Subsystem2/1(Out1) -> Merge1/10
  If1/8 -> If Action Subsystem1/Action
  If Action Subsystem3/1(Out1) -> Merge1/7
  If1/6 -> If Action Subsystem4/Action
  From Workspace2/1 -> If1/1
  Merge1/1 -> Out1/1
  If Action Subsystem6/1(Out1) -> Merge1/5
  If Action Subsystem7/1(Out1) -> Merge1/3
  If1/9 -> If Action Subsystem10/Action
  If Action Subsystem10/1(Out1) -> Merge1/9

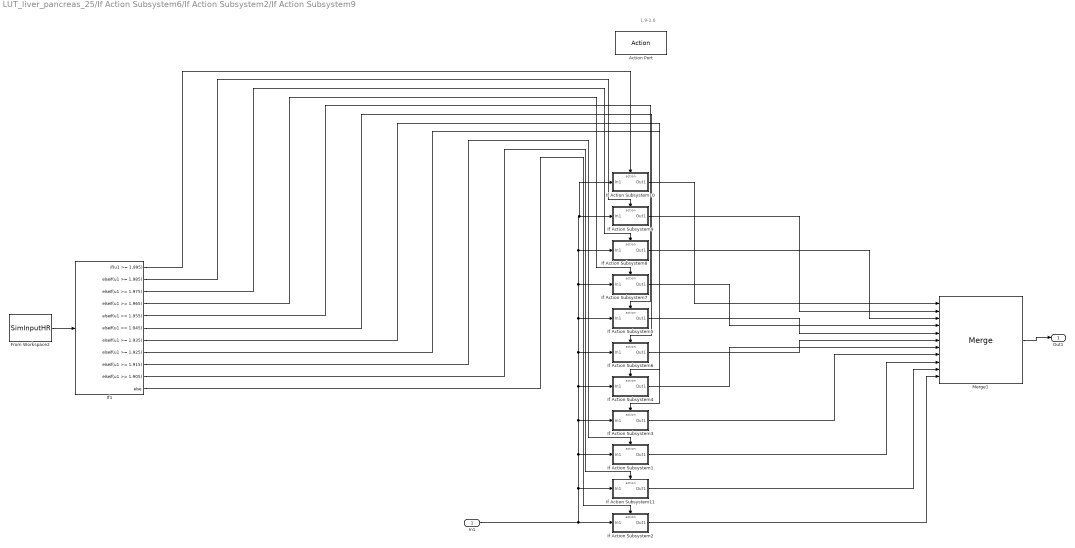
== system LUT_liver_pancreas_25/If Action Subsystem6/If Action Subsystem2/If Action Subsystem9 ==
  note: 1.9-2.0
  In1 : Inport
  Action Port : ActionPort  ActionPortLabel=if(u1 >= 1.895)
  From Workspace2 : FromWorkspace  VariableName=SimInputHR  Interpolate=off  OutputAfterFinalValue=Setting to zero
  If Action Subsystem1 : Subsystem  TreatAsAtomicUnit=on
  If Action Subsystem10 : Subsystem  TreatAsAtomicUnit=on
  If Action Subsystem11 : Subsystem  TreatAsAtomicUnit=on
  If Action Subsystem2 : Subsystem  TreatAsAtomicUnit=on
  If Action Subsystem3 : Subsystem  TreatAsAtomicUnit=on
  If Action Subsystem4 : Subsystem  TreatAsAtomicUnit=on
  If Action Subsystem5 : Subsystem  TreatAsAtomicUnit=on
  If Action Subsystem6 : Subsystem  TreatAsAtomicUnit=on
  If Action Subsystem7 : Subsystem  TreatAsAtomicUnit=on
  If Action Subsystem8 : Subsystem  TreatAsAtomicUnit=on
  If Action Subsystem9 : Subsystem  TreatAsAtomicUnit=on
  If1 : If  IfExpression=u1 >= 1.995  ElseIfExpressions=u1 >= 1.985, u1 >= 1.975, u1 >= 1.965, u1 >= 1.955, u1 >= 1.945, u1 >= 1.935, u1 >= 1.925, u1 >= 1.915, u1 >= 1.905
  Merge1 : Merge  Inputs=11
  Out1 : Outport
  wires:
  Merge1/1 -> Out1/1
  From Workspace2/1 -> If1/1
  If1/2 -> If Action Subsystem9/Action
  If1/3 -> If Action Subsystem8/Action
  If1/4 -> If Action Subsystem7/Action
  If1/5 -> If Action Subsystem5/Action
  If1/6 -> If Action Subsystem6/Action
  If1/7 -> If Action Subsystem4/Action
  If1/8 -> If Action Subsystem3/Action
  If1/9 -> If Action Subsystem1/Action
  If1/11 -> If Action Subsystem2/Action
  If Action Subsystem9/1(Out1) -> Merge1/2
  If Action Subsystem8/1(Out1) -> Merge1/3
  If Action Subsystem7/1(Out1) -> Merge1/4
  If Action Subsystem5/1(Out1) -> Merge1/5
  If Action Subsystem6/1(Out1) -> Merge1/6
  If Action Subsystem4/1(Out1) -> Merge1/7
  If Action Subsystem3/1(Out1) -> Merge1/8
  If Action Subsystem2/1(Out1) -> Merge1/11
  If Action Subsystem1/1(Out1) -> Merge1/9
  In1/1 -> If Action Subsystem1/1(In1), If Action Subsystem3/1(In1), If Action Subsystem4/1(In1), If Action Subsystem7/1(In1), If Action Subsystem8/1(In1), If Action Subsystem10/1(In1), If Action Subsystem9/1(In1), If Action Subsystem5/1(In1), If Action Subsystem6/1(In1), If Action Subsystem11/1(In1), If Action Subsystem2/1(In1)
  If1/1 -> If Action Subsystem10/Action
  If Action Subsystem10/1(Out1) -> Merge1/1
  If1/10 -> If Action Subsystem11/Action
  If Action Subsystem11/1(Out1) -> Merge1/10

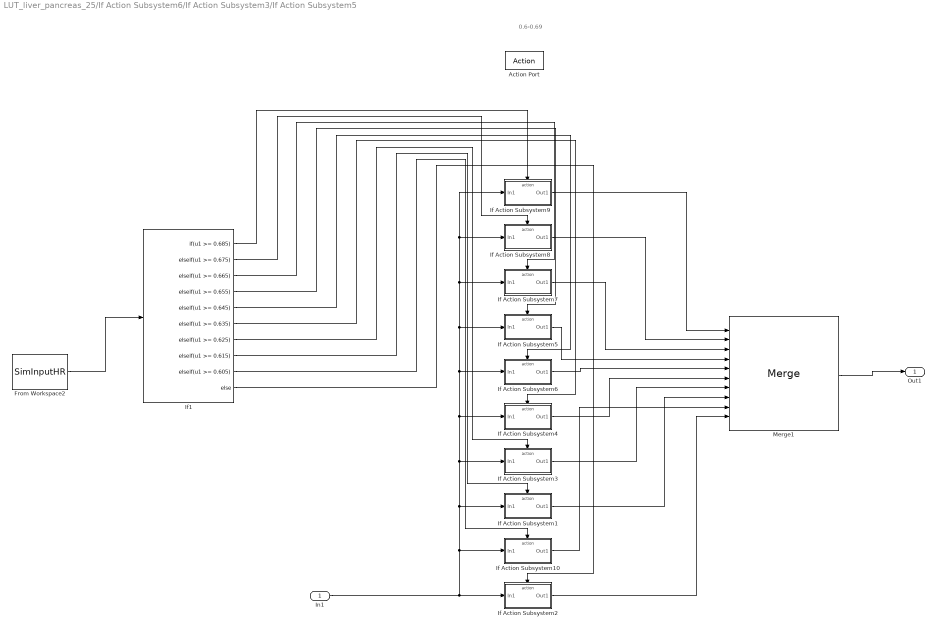
== system LUT_liver_pancreas_25/If Action Subsystem6/If Action Subsystem3/If Action Subsystem5 ==
  note: 0.6-0.69
  In1 : Inport
  Action Port : ActionPort  ActionPortLabel=elseif( u1 >= 0595)
  From Workspace2 : FromWorkspace  VariableName=SimInputHR  Interpolate=off  OutputAfterFinalValue=Setting to zero
  If Action Subsystem1 : Subsystem  TreatAsAtomicUnit=on
  If Action Subsystem10 : Subsystem  TreatAsAtomicUnit=on
  If Action Subsystem2 : Subsystem  TreatAsAtomicUnit=on
  If Action Subsystem3 : Subsystem  TreatAsAtomicUnit=on
  If Action Subsystem4 : Subsystem  TreatAsAtomicUnit=on
  If Action Subsystem5 : Subsystem  TreatAsAtomicUnit=on
  If Action Subsystem6 : Subsystem  TreatAsAtomicUnit=on
  If Action Subsystem7 : Subsystem  TreatAsAtomicUnit=on
  If Action Subsystem8 : Subsystem  TreatAsAtomicUnit=on
  If Action Subsystem9 : Subsystem  TreatAsAtomicUnit=on
  If1 : If  IfExpression=u1 >= 0.685  ElseIfExpressions=u1 >= 0.675, u1 >= 0.665, u1 >= 0.655, u1 >= 0.645, u1 >= 0.635, u1 >= 0.625, u1 >= 0.615, u1 >= 0.605
  Merge1 : Merge  Inputs=10
  Out1 : Outport
  wires:
  If1/10 -> If Action Subsystem2/Action
  If Action Subsystem4/1(Out1) -> Merge1/6
  From Workspace2/1 -> If1/1
  If Action Subsystem6/1(Out1) -> Merge1/5
  Merge1/1 -> Out1/1
  If1/8 -> If Action Subsystem1/Action
  If Action Subsystem3/1(Out1) -> Merge1/7
  In1/1 -> If Action Subsystem1/1(In1), If Action Subsystem3/1(In1), If Action Subsystem4/1(In1), If Action Subsystem7/1(In1), If Action Subsystem8/1(In1), If Action Subsystem9/1(In1), If Action Subsystem5/1(In1), If Action Subsystem6/1(In1), If Action Subsystem10/1(In1), If Action Subsystem2/1(In1)
  If1/6 -> If Action Subsystem4/Action
  If Action Subsystem1/1(Out1) -> Merge1/8
  If1/4 -> If Action Subsystem5/Action
  If Action Subsystem8/1(Out1) -> Merge1/2
  If1/5 -> If Action Subsystem6/Action
  If Action Subsystem7/1(Out1) -> Merge1/3
  If1/3 -> If Action Subsystem7/Action
  If1/7 -> If Action Subsystem3/Action
  If Action Subsystem5/1(Out1) -> Merge1/4
  If Action Subsystem2/1(Out1) -> Merge1/10
  If1/2 -> If Action Subsystem8/Action
  If1/1 -> If Action Subsystem9/Action
  If Action Subsystem9/1(Out1) -> Merge1/1
  If Action Subsystem10/1(Out1) -> Merge1/9
  If1/9 -> If Action Subsystem10/Action

== system LUT_liver_pancreas_25/If Action Subsystem6/If Action Subsystem3/If Action Subsystem6 ==
  note: 0.5-0.59
  In1 : Inport
  Action Port : ActionPort  ActionPortLabel=else
  From Workspace2 : FromWorkspace  VariableName=SimInputHR  Interpolate=off  OutputAfterFinalValue=Setting to zero
  If Action Subsystem1 : Subsystem  TreatAsAtomicUnit=on
  If Action Subsystem10 : Subsystem  TreatAsAtomicUnit=on
  If Action Subsystem2 : Subsystem  TreatAsAtomicUnit=on
  If Action Subsystem3 : Subsystem  TreatAsAtomicUnit=on
  If Action Subsystem4 : Subsystem  TreatAsAtomicUnit=on
  If Action Subsystem5 : Subsystem  TreatAsAtomicUnit=on
  If Action Subsystem6 : Subsystem  TreatAsAtomicUnit=on
  If Action Subsystem7 : Subsystem  TreatAsAtomicUnit=on
  If Action Subsystem8 : Subsystem  TreatAsAtomicUnit=on
  If Action Subsystem9 : Subsystem  TreatAsAtomicUnit=on
  If1 : If  IfExpression=u1 >= 0.585  ElseIfExpressions=u1 >= 0.575, u1 >= 0.565, u1 >= 0.555, u1 >= 0.545, u1 >= 0.535, u1 >= 0.525, u1 >= 0.515, u1 >= 0.505
  Merge1 : Merge  Inputs=10
  Out1 : Outport
  wires:
  If1/10 -> If Action Subsystem2/Action
  If Action Subsystem4/1(Out1) -> Merge1/6
  From Workspace2/1 -> If1/1
  If Action Subsystem6/1(Out1) -> Merge1/5
  Merge1/1 -> Out1/1
  If1/8 -> If Action Subsystem1/Action
  If Action Subsystem3/1(Out1) -> Merge1/7
  In1/1 -> If Action Subsystem1/1(In1), If Action Subsystem3/1(In1), If Action Subsystem4/1(In1), If Action Subsystem7/1(In1), If Action Subsystem8/1(In1), If Action Subsystem9/1(In1), If Action Subsystem5/1(In1), If Action Subsystem6/1(In1), If Action Subsystem10/1(In1), If Action Subsystem2/1(In1)
  If1/6 -> If Action Subsystem4/Action
  If Action Subsystem1/1(Out1) -> Merge1/8
  If1/4 -> If Action Subsystem5/Action
  If Action Subsystem8/1(Out1) -> Merge1/2
  If1/5 -> If Action Subsystem6/Action
  If Action Subsystem7/1(Out1) -> Merge1/3
  If1/3 -> If Action Subsystem7/Action
  If1/7 -> If Action Subsystem3/Action
  If Action Subsystem5/1(Out1) -> Merge1/4
  If Action Subsystem2/1(Out1) -> Merge1/10
  If1/2 -> If Action Subsystem8/Action
  If1/1 -> If Action Subsystem9/Action
  If Action Subsystem9/1(Out1) -> Merge1/1
  If Action Subsystem10/1(Out1) -> Merge1/9
  If1/9 -> If Action Subsystem10/Action

== system LUT_liver_pancreas_25/If Action Subsystem6/If Action Subsystem3/If Action Subsystem7 ==
  note: 0.7-0.79
  In1 : Inport
  Action Port : ActionPort  ActionPortLabel=elseif( u1 >= 0.695)
  From Workspace2 : FromWorkspace  VariableName=SimInputHR  Interpolate=off  OutputAfterFinalValue=Setting to zero
  If Action Subsystem1 : Subsystem  TreatAsAtomicUnit=on
  If Action Subsystem10 : Subsystem  TreatAsAtomicUnit=on
  If Action Subsystem2 : Subsystem  TreatAsAtomicUnit=on
  If Action Subsystem3 : Subsystem  TreatAsAtomicUnit=on
  If Action Subsystem4 : Subsystem  TreatAsAtomicUnit=on
  If Action Subsystem5 : Subsystem  TreatAsAtomicUnit=on
  If Action Subsystem6 : Subsystem  TreatAsAtomicUnit=on
  If Action Subsystem7 : Subsystem  TreatAsAtomicUnit=on
  If Action Subsystem8 : Subsystem  TreatAsAtomicUnit=on
  If Action Subsystem9 : Subsystem  TreatAsAtomicUnit=on
  If1 : If  IfExpression=u1 >= 0.785  ElseIfExpressions=u1 >= 0.775, u1 >= 0.765, u1 >= 0.755, u1 >= 0.745, u1 >= 0.735, u1 >= 0.725, u1 >= 0.715, u1 >= 0.705
  Merge1 : Merge  Inputs=10
  Out1 : Outport
  wires:
  If1/10 -> If Action Subsystem2/Action
  If Action Subsystem4/1(Out1) -> Merge1/6
  From Workspace2/1 -> If1/1
  If Action Subsystem6/1(Out1) -> Merge1/5
  Merge1/1 -> Out1/1
  If1/8 -> If Action Subsystem1/Action
  If Action Subsystem3/1(Out1) -> Merge1/7
  In1/1 -> If Action Subsystem1/1(In1), If Action Subsystem3/1(In1), If Action Subsystem4/1(In1), If Action Subsystem7/1(In1), If Action Subsystem8/1(In1), If Action Subsystem9/1(In1), If Action Subsystem5/1(In1), If Action Subsystem6/1(In1), If Action Subsystem10/1(In1), If Action Subsystem2/1(In1)
  If1/6 -> If Action Subsystem4/Action
  If Action Subsystem1/1(Out1) -> Merge1/8
  If1/4 -> If Action Subsystem5/Action
  If Action Subsystem8/1(Out1) -> Merge1/2
  If1/5 -> If Action Subsystem6/Action
  If Action Subsystem7/1(Out1) -> Merge1/3
  If1/3 -> If Action Subsystem7/Action
  If1/7 -> If Action Subsystem3/Action
  If Action Subsystem5/1(Out1) -> Merge1/4
  If Action Subsystem2/1(Out1) -> Merge1/10
  If1/2 -> If Action Subsystem8/Action
  If1/1 -> If Action Subsystem9/Action
  If Action Subsystem9/1(Out1) -> Merge1/1
  If1/9 -> If Action Subsystem10/Action
  If Action Subsystem10/1(Out1) -> Merge1/9

== system LUT_liver_pancreas_25/If Action Subsystem6/If Action Subsystem3/If Action Subsystem8 ==
  note: 0.8-0.89
  In1 : Inport
  Action Port : ActionPort  ActionPortLabel=elseif(u1 >= 0.795)
  From Workspace2 : FromWorkspace  VariableName=SimInputHR  Interpolate=off  OutputAfterFinalValue=Setting to zero
  If Action Subsystem1 : Subsystem  TreatAsAtomicUnit=on
  If Action Subsystem10 : Subsystem  TreatAsAtomicUnit=on
  If Action Subsystem2 : Subsystem  TreatAsAtomicUnit=on
  If Action Subsystem3 : Subsystem  TreatAsAtomicUnit=on
  If Action Subsystem4 : Subsystem  TreatAsAtomicUnit=on
  If Action Subsystem5 : Subsystem  TreatAsAtomicUnit=on
  If Action Subsystem6 : Subsystem  TreatAsAtomicUnit=on
  If Action Subsystem7 : Subsystem  TreatAsAtomicUnit=on
  If Action Subsystem8 : Subsystem  TreatAsAtomicUnit=on
  If Action Subsystem9 : Subsystem  TreatAsAtomicUnit=on
  If1 : If  IfExpression=u1 >= 0.885  ElseIfExpressions=u1 >= 0.875, u1 >= 0.865, u1 >= 0.855, u1 >= 0.845, u1 >= 0.835, u1 >= 0.825, u1 >= 0.815, u1 >= 0.805
  Merge1 : Merge  Inputs=10
  Out1 : Outport
  wires:
  If1/10 -> If Action Subsystem2/Action
  If Action Subsystem4/1(Out1) -> Merge1/6
  From Workspace2/1 -> If1/1
  If Action Subsystem6/1(Out1) -> Merge1/5
  Merge1/1 -> Out1/1
  If1/8 -> If Action Subsystem1/Action
  If Action Subsystem3/1(Out1) -> Merge1/7
  In1/1 -> If Action Subsystem1/1(In1), If Action Subsystem3/1(In1), If Action Subsystem4/1(In1), If Action Subsystem7/1(In1), If Action Subsystem8/1(In1), If Action Subsystem9/1(In1), If Action Subsystem5/1(In1), If Action Subsystem6/1(In1), If Action Subsystem10/1(In1), If Action Subsystem2/1(In1)
  If1/6 -> If Action Subsystem4/Action
  If Action Subsystem1/1(Out1) -> Merge1/8
  If1/4 -> If Action Subsystem5/Action
  If Action Subsystem8/1(Out1) -> Merge1/2
  If1/5 -> If Action Subsystem6/Action
  If Action Subsystem7/1(Out1) -> Merge1/3
  If1/3 -> If Action Subsystem7/Action
  If1/7 -> If Action Subsystem3/Action
  If Action Subsystem5/1(Out1) -> Merge1/4
  If Action Subsystem2/1(Out1) -> Merge1/10
  If1/2 -> If Action Subsystem8/Action
  If1/1 -> If Action Subsystem9/Action
  If Action Subsystem9/1(Out1) -> Merge1/1
  If1/9 -> If Action Subsystem10/Action
  If Action Subsystem10/1(Out1) -> Merge1/9

== system LUT_liver_pancreas_25/If Action Subsystem6/If Action Subsystem3/If Action Subsystem9 ==
  note: 0.9-0.99
  In2 : Inport
  Action Port : ActionPort  ActionPortLabel=if(u1 >= 0.895)
  From Workspace2 : FromWorkspace  VariableName=SimInputHR  Interpolate=off  OutputAfterFinalValue=Setting to zero
  If Action Subsystem1 : Subsystem  TreatAsAtomicUnit=on
  If Action Subsystem10 : Subsystem  TreatAsAtomicUnit=on
  If Action Subsystem2 : Subsystem  TreatAsAtomicUnit=on
  If Action Subsystem3 : Subsystem  TreatAsAtomicUnit=on
  If Action Subsystem4 : Subsystem  TreatAsAtomicUnit=on
  If Action Subsystem5 : Subsystem  TreatAsAtomicUnit=on
  If Action Subsystem6 : Subsystem  TreatAsAtomicUnit=on
  If Action Subsystem7 : Subsystem  TreatAsAtomicUnit=on
  If Action Subsystem8 : Subsystem  TreatAsAtomicUnit=on
  If Action Subsystem9 : Subsystem  TreatAsAtomicUnit=on
  If1 : If  IfExpression=u1 >= 0.985  ElseIfExpressions=u1 >= 0.975, u1 >= 0.965, u1 >= 0.955, u1 >= 0.945, u1 >= 0.935, u1 >= 0.925, u1 >= 0.915, u1 >= 0.905
  Merge1 : Merge  Inputs=10
  Out2 : Outport
  wires:
  If1/10 -> If Action Subsystem2/Action
  If Action Subsystem4/1(Out1) -> Merge1/6
  From Workspace2/1 -> If1/1
  If Action Subsystem6/1(Out1) -> Merge1/5
  Merge1/1 -> Out2/1
  If1/8 -> If Action Subsystem1/Action
  If Action Subsystem3/1(Out1) -> Merge1/7
  In2/1 -> If Action Subsystem10/1(In1), If Action Subsystem1/1(In1), If Action Subsystem3/1(In1), If Action Subsystem4/1(In1), If Action Subsystem7/1(In1), If Action Subsystem8/1(In1), If Action Subsystem9/1(In1), If Action Subsystem5/1(In1), If Action Subsystem6/1(In1), If Action Subsystem2/1(In1)
  If1/6 -> If Action Subsystem4/Action
  If Action Subsystem1/1(Out1) -> Merge1/8
  If1/4 -> If Action Subsystem5/Action
  If Action Subsystem8/1(Out1) -> Merge1/2
  If1/5 -> If Action Subsystem6/Action
  If Action Subsystem7/1(Out1) -> Merge1/3
  If1/3 -> If Action Subsystem7/Action
  If1/7 -> If Action Subsystem3/Action
  If Action Subsystem5/1(Out1) -> Merge1/4
  If Action Subsystem2/1(Out1) -> Merge1/10
  If1/2 -> If Action Subsystem8/Action
  If1/1 -> If Action Subsystem9/Action
  If Action Subsystem9/1(Out1) -> Merge1/1
  If1/9 -> If Action Subsystem10/Action
  If Action Subsystem10/1(Out1) -> Merge1/9

== system LUT_liver_pancreas_25/If Action Subsystem6/If Action Subsystem1/If Action Subsystem5/If Action Subsystem1 ==
  In1 : Inport
  Action Port : ActionPort  ActionPortLabel=elseif( u1 >= 1.115)
  LUT 1.12RR : Lookup_n-D  NumberOfTableDimensions=1  BreakpointsForDimension1=[402.3432;510.8916;609.2833;707.7954;806.2198;904.5642;1002.848;1101.089;1199.296;1297.479;1395.643;1493.792;1591.929;1690.056;1788.173;1886.28;1984.374]  Table=[400;500;600;700;800;900;1000;1100;1200;1300;1400;1500;1600;1700;1800;1900;2000]  InternalRulePriority=Speed  RndMeth=Simplest
  Out1 : Outport
  wires:
  In1/1 -> LUT 1.12RR/1
  LUT 1.12RR/1 -> Out1/1

== system LUT_liver_pancreas_25/If Action Subsystem6/If Action Subsystem1/If Action Subsystem5/If Action Subsystem10 ==
  In1 : Inport
  Action Port : ActionPort  ActionPortLabel=elseif( u1 >= 1.105)
  LUT 1.11RR : Lookup_n-D  NumberOfTableDimensions=1  BreakpointsForDimension1=[402.4254;511.03;609.4791;708.0554;806.5484;904.9641;1003.322;1101.636;1199.919;1298.179;1396.419;1494.646;1592.86;1691.064;1789.259;1887.444;1985.614]  Table=[400;500;600;700;800;900;1000;1100;1200;1300;1400;1500;1600;1700;1800;1900;2000]  InternalRulePriority=Speed  RndMeth=Simplest
  Out1 : Outport
  wires:
  In1/1 -> LUT 1.11RR/1
  LUT 1.11RR/1 -> Out1/1

== system LUT_liver_pancreas_25/If Action Subsystem6/If Action Subsystem1/If Action Subsystem5/If Action Subsystem2 ==
  In1 : Inport
  Action Port : ActionPort  ActionPortLabel=else
  LUT 1.10RR : Lookup_n-D  NumberOfTableDimensions=1  BreakpointsForDimension1=[402.5094;511.172;609.6799;708.3222;806.8853;905.3738;1003.806;1102.197;1200.557;1298.894;1397.213;1495.518;1593.811;1692.095;1790.369;1888.633;1986.88]  Table=[400;500;600;700;800;900;1000;1100;1200;1300;1400;1500;1600;1700;1800;1900;2000]  InternalRulePriority=Speed  RndMeth=Simplest
  Out1 : Outport
  wires:
  In1/1 -> LUT 1.10RR/1
  LUT 1.10RR/1 -> Out1/1

== system LUT_liver_pancreas_25/If Action Subsystem6/If Action Subsystem1/If Action Subsystem5/If Action Subsystem3 ==
  In1 : Inport
  Action Port : ActionPort  ActionPortLabel=elseif( u1 >= 1.125)
  LUT 1.13RR : Lookup_n-D  NumberOfTableDimensions=1  BreakpointsForDimension1=[402.2628;510.7566;609.0925;707.5418;805.8992;904.1738;1002.386;1100.554;1198.687;1296.796;1394.885;1492.958;1591.019;1689.069;1787.11;1885.141;1983.16]  Table=[400;500;600;700;800;900;1000;1100;1200;1300;1400;1500;1600;1700;1800;1900;2000]  InternalRulePriority=Speed  RndMeth=Simplest
  Out1 : Outport
  wires:
  In1/1 -> LUT 1.13RR/1
  LUT 1.13RR/1 -> Out1/1

== system LUT_liver_pancreas_25/If Action Subsystem6/If Action Subsystem1/If Action Subsystem5/If Action Subsystem4 ==
  In1 : Inport
  Action Port : ActionPort  ActionPortLabel=elseif( u1 >= 1.135)
  LUT 1.14RR : Lookup_n-D  NumberOfTableDimensions=1  BreakpointsForDimension1=[402.1842;510.6248;608.9064;707.2944;805.5863;903.7926;1001.935;1100.031;1198.092;1296.127;1394.142;1492.142;1590.128;1688.104;1786.07;1884.026;1981.971]  Table=[400;500;600;700;800;900;1000;1100;1200;1300;1400;1500;1600;1700;1800;1900;2000]  InternalRulePriority=Speed  RndMeth=Simplest
  Out1 : Outport
  wires:
  In1/1 -> LUT 1.14RR/1
  LUT 1.14RR/1 -> Out1/1

== system LUT_liver_pancreas_25/If Action Subsystem6/If Action Subsystem1/If Action Subsystem5/If Action Subsystem5 ==
  In1 : Inport
  Action Port : ActionPort  ActionPortLabel=elseif( u1 >= 1.155)
  LUT 1.16RR : Lookup_n-D  NumberOfTableDimensions=1  BreakpointsForDimension1=[402.0318;510.3708;608.5479;706.8176;804.9828;903.0568;1001.063;1099.02;1196.941;1294.834;1392.706;1490.561;1588.403;1686.233;1784.054;1881.865;1979.665]  Table=[400;500;600;700;800;900;1000;1100;1200;1300;1400;1500;1600;1700;1800;1900;2000]  InternalRulePriority=Speed  RndMeth=Simplest
  Out1 : Outport
  wires:
  In1/1 -> LUT 1.16RR/1
  LUT 1.16RR/1 -> Out1/1

== system LUT_liver_pancreas_25/If Action Subsystem6/If Action Subsystem1/If Action Subsystem5/If Action Subsystem6 ==
  In1 : Inport
  Action Port : ActionPort  ActionPortLabel=elseif( u1 >= 1.145)
  LUT 1.15RR : Lookup_n-D  NumberOfTableDimensions=1  BreakpointsForDimension1=[402.1072;510.4963;608.725;707.0531;805.2809;903.4204;1001.494;1099.52;1197.51;1295.473;1393.416;1491.343;1589.256;1687.159;1785.051;1882.934;1980.806]  Table=[400;500;600;700;800;900;1000;1100;1200;1300;1400;1500;1600;1700;1800;1900;2000]  InternalRulePriority=Speed  RndMeth=Simplest
  Out1 : Outport
  wires:
  In1/1 -> LUT 1.15RR/1
  LUT 1.15RR/1 -> Out1/1

== system LUT_liver_pancreas_25/If Action Subsystem6/If Action Subsystem1/If Action Subsystem5/If Action Subsystem7 ==
  In1 : Inport
  Action Port : ActionPort  ActionPortLabel=elseif( u1 >= 1.165)
  LUT 1.17RR : Lookup_n-D  NumberOfTableDimensions=1  BreakpointsForDimension1=[401.9578;510.2483;608.3752;706.5878;804.6917;902.7017;1000.642;1098.532;1196.384;1294.208;1392.01;1489.796;1587.567;1685.327;1783.077;1880.817;1978.547]  Table=[400;500;600;700;800;900;1000;1100;1200;1300;1400;1500;1600;1700;1800;1900;2000]  InternalRulePriority=Speed  RndMeth=Simplest
  Out1 : Outport
  wires:
  In1/1 -> LUT 1.17RR/1
  LUT 1.17RR/1 -> Out1/1

== system LUT_liver_pancreas_25/If Action Subsystem6/If Action Subsystem1/If Action Subsystem5/If Action Subsystem8 ==
  In1 : Inport
  Action Port : ActionPort  ActionPortLabel=elseif(u1 >= 1.175)
  LUT 1.18RR : Lookup_n-D  NumberOfTableDimensions=1  BreakpointsForDimension1=[401.8854;510.1287;608.2066;706.3635;804.4074;902.3547;1000.231;1098.054;1195.84;1293.596;1391.33;1489.046;1586.749;1684.44;1782.12;1879.791;1977.452]  Table=[400;500;600;700;800;900;1000;1100;1200;1300;1400;1500;1600;1700;1800;1900;2000]  InternalRulePriority=Speed  RndMeth=Simplest
  Out1 : Outport
  wires:
  In1/1 -> LUT 1.18RR/1
  LUT 1.18RR/1 -> Out1/1

== system LUT_liver_pancreas_25/If Action Subsystem6/If Action Subsystem1/If Action Subsystem5/If Action Subsystem9 ==
  In1 : Inport
  Action Port : ActionPort  ActionPortLabel=if(u1 >= 1.185)
  LUT 1.19RR : Lookup_n-D  NumberOfTableDimensions=1  BreakpointsForDimension1=[401.8144;510.0117;608.042;706.1445;804.1298;902.0156;999.8281;1097.587;1195.307;1292.997;1390.664;1488.313;1585.948;1683.57;1781.183;1878.785;1976.378]  Table=[400;500;600;700;800;900;1000;1100;1200;1300;1400;1500;1600;1700;1800;1900;2000]  InternalRulePriority=Speed  RndMeth=Simplest
  Out1 : Outport
  wires:
  In1/1 -> LUT 1.19RR/1
  LUT 1.19RR/1 -> Out1/1

== system LUT_liver_pancreas_25/If Action Subsystem6/If Action Subsystem1/If Action Subsystem6/If Action Subsystem1 ==
  In1 : Inport
  Action Port : ActionPort  ActionPortLabel=elseif( u1 >= 1.015)
  LUT 1.02RR : Lookup_n-D  NumberOfTableDimensions=1  BreakpointsForDimension1=[403.2604;512.4553;611.496;710.7287;809.9161;909.0507;1008.144;1107.206;1206.244;1305.266;1404.274;1503.271;1602.26;1701.24;1800.21;1899.163;1998.054]  Table=[400;500;600;700;800;900;1000;1100;1200;1300;1400;1500;1600;1700;1800;1900;2000]  InternalRulePriority=Speed  RndMeth=Simplest
  Out1 : Outport
  wires:
  In1/1 -> LUT 1.02RR/1
  LUT 1.02RR/1 -> Out1/1

== system LUT_liver_pancreas_25/If Action Subsystem6/If Action Subsystem1/If Action Subsystem6/If Action Subsystem10 ==
  In1 : Inport
  Action Port : ActionPort  ActionPortLabel=elseif( u1 >= 1.005)
  LUT 1.01RR : Lookup_n-D  NumberOfTableDimensions=1  BreakpointsForDimension1=[403.3658;512.6369;611.7529;711.0682;810.3426;909.5667;1008.751;1107.905;1207.038;1306.153;1405.256;1504.349;1603.433;1702.509;1801.575;1900.621;1999.585]  Table=[400;500;600;700;800;900;1000;1100;1200;1300;1400;1500;1600;1700;1800;1900;2000]  InternalRulePriority=Speed  RndMeth=Simplest
  Out1 : Outport
  wires:
  In1/1 -> LUT 1.01RR/1
  LUT 1.01RR/1 -> Out1/1

== system LUT_liver_pancreas_25/If Action Subsystem6/If Action Subsystem1/If Action Subsystem6/If Action Subsystem2 ==
  In1 : Inport
  Action Port : ActionPort  ActionPortLabel=else
  LUT 1.00RR : Lookup_n-D  NumberOfTableDimensions=1  BreakpointsForDimension1=[403.4742;512.824;612.0175;711.4176;810.781;910.0968;1009.375;1108.624;1207.852;1307.064;1406.264;1505.454;1604.636;1703.811;1802.974;1902.114;2001.141]  Table=[400;500;600;700;800;900;1000;1100;1200;1300;1400;1500;1600;1700;1800;1900;2000]  InternalRulePriority=Speed  RndMeth=Simplest
  Out1 : Outport
  wires:
  In1/1 -> LUT 1.00RR/1
  LUT 1.00RR/1 -> Out1/1
